simulink model "sampleModel7"  (R2021a)
settings: Solver=VariableStepAuto  StartTime=0.0  StopTime=10.0  RelTol=1e-3
undefined symbols (not defined in the file): DiscIntNeverNeededParam, magnitude, Newton, Raphson
libraries: simulink x210, pid_lib x47, simulink_need_slupdate x2
(part 5 of 8)

== system sampleModel7/cfblk409/cfblk12 ==
  cfblk1 : Inport
  cfblk11 : Inport  Port=2
  cfblk12 : Inport  Port=3
  cfblk13 : Inport  Port=4
  cfblk14 : Inport  Port=5
  cfblk10 : Constant  Value=[285971004.246024]  SampleTime=1
  cfblk3 : Delay  ShowEnablePort=on
      settings: InputPortMap=u0,e6
  cfblk4 : simulink/Discrete/Transfer Fcn Lead or Lag  PoleZ=0.95  ZeroZ=0.75  ICPrevOutput=0.0  ICPrevInput=0.0  DoSatur=off
      settings: SourceProductBaseCode=SL
  cfblk5 : Sum  Inputs=-+
  cfblk6 : MinMax  Function=max  Inputs=3
  cfblk7 : Rounding
  cfblk8 : Constant  Value=[956433965.581636]  SampleTime=1
  cfblk9 : Constant  Value=[825464940.183947]  SampleTime=1
  cfblk2 : Outport
  cfblk15 : Outport  Port=2
  wires:
  cfblk1/1 -> cfblk5/1
  cfblk12/1 -> cfblk15/1
  cfblk10/1 -> cfblk6/1
  cfblk7/1 -> cfblk5/2
  cfblk14/1 -> cfblk6/2
  cfblk13/1 -> cfblk6/3
  cfblk11/1 -> cfblk7/1
  cfblk9/1 -> cfblk3/1
  cfblk6/1 -> cfblk4/1
  cfblk5/1 -> cfblk3/2
  cfblk3/1 -> cfblk2/1

== system sampleModel7/cfblk410/cfblk6 ==
  cfblk1 : Inport
  cfblk9 : Inport  Port=2
  cfblk10 : Inport  Port=3
  cfblk11 : Inport  Port=4
  cfblk12 : Inport  Port=5
  cfblk3 : Product  Inputs=**
  cfblk4 : MinMax  Inputs=2
  cfblk5 : DotProduct  InputSameDT=on  OutDataTypeStr=Inherit: Inherit via internal rule
  cfblk6 : Constant  Value=[-599214719.429077]  SampleTime=1
  cfblk7 : Subsystem
  cfblk8 : Subsystem
  cfblk2 : Outport
  wires:
  cfblk11/1 -> cfblk5/1
  cfblk7/1(cfblk2) -> cfblk5/2
  cfblk5/1 -> cfblk8/1(cfblk1)
  cfblk6/1 -> cfblk2/1
  cfblk10/1 -> cfblk7/1(cfblk1), cfblk4/2
  cfblk3/1 -> cfblk7/2(cfblk13)
  cfblk9/1 -> cfblk3/1
  cfblk1/1 -> cfblk3/2
  cfblk12/1 -> cfblk8/2(cfblk7)
  cfblk8/1(cfblk2) -> cfblk4/1

== system sampleModel7/cfblk412/cfblk11 ==
  cfblk1 : Inport
  cfblk7 : Inport  Port=2
  cfblk8 : Inport  Port=3
  cfblk9 : Inport  Port=4
  cfblk3 : DiscreteFir
  cfblk4 : Sum  Inputs=|++
  cfblk5 : Rounding
  cfblk6 : Subsystem
  cfblk2 : Outport
  wires:
  cfblk3/1 -> cfblk4/1
  cfblk6/1(cfblk2) -> cfblk2/1
  cfblk8/1 -> cfblk4/2
  cfblk7/1 -> cfblk3/1
  cfblk5/1 -> cfblk6/1(cfblk1)
  cfblk1/1 -> cfblk6/2(cfblk12)
  cfblk9/1 -> cfblk5/1

== system sampleModel7/cfblk412/cfblk12 ==
  cfblk1 : Inport
  cfblk5 : Inport  Port=2
  cfblk6 : Inport  Port=3
  cfblk7 : Inport  Port=4
  cfblk8 : Inport  Port=5
  cfblk3 : simulink/Discrete/Tapped Delay  vinit=0.0  samptime=-1  NumDelays=1  DelayOrder=Oldest  includeCurrent=off
  cfblk4 : Gain  Gain=[760831877.903095]
  cfblk2 : Outport
  wires:
  cfblk1/1 -> cfblk3/1
  cfblk7/1 -> cfblk4/1
  cfblk3/1 -> cfblk2/1

== system sampleModel7/cfblk413/cfblk7 ==
  cfblk1 : Inport
  cfblk7 : Inport  Port=2
  cfblk8 : Inport  Port=3
  cfblk9 : Inport  Port=4
  cfblk10 : Inport  Port=5
  cfblk11 : Inport  Port=6
  cfblk12 : Inport  Port=7
  cfblk13 : Inport  Port=8
  cfblk3 : ComplexToRealImag
  cfblk4 : Gain  Gain=[-505145990.047614]
  cfblk5 : Product  Inputs=**
  cfblk6 : Assignment  DiagnosticForDimensions=Warning  IndexOptions=Index vector (dialog)  Indices=1  OutputSizes=1
  cfblk2 : Outport
  cfblk14 : Outport  Port=2
  wires:
  cfblk6/1 -> cfblk14/1
  cfblk11/1 -> cfblk3/1
  cfblk5/1 -> cfblk4/1
  cfblk9/1 -> cfblk5/1
  cfblk12/1 -> cfblk2/1
  cfblk3/1 -> cfblk6/1
  cfblk1/1 -> cfblk5/2
  cfblk8/1 -> cfblk6/2

== system sampleModel7/cfblk414/cfblk8 ==
  cfblk1 : Inport
  cfblk10 : Inport  Port=2
  cfblk11 : Inport  Port=3
  cfblk12 : Inport  Port=4
  cfblk13 : Inport  Port=5
  cfblk15 : Delay
  cfblk3 : DiscreteFir
  cfblk4 : Sum  Inputs=+
  cfblk5 : Product
  cfblk6 : Constant  Value=[-301322908.390573]  SampleTime=1
  cfblk7 : Constant  Value=[-743268385.761539]  SampleTime=1
  cfblk8 : Constant  Value=[952161668.056087]  SampleTime=1
  cfblk9 : Constant  Value=[508901382.821117]  SampleTime=1
  cfblk2 : Outport
  cfblk14 : Outport  Port=2
  wires:
  cfblk7/1 -> cfblk2/1
  cfblk9/1 -> cfblk14/1
  cfblk6/1 -> cfblk5/1
  cfblk3/1 -> cfblk5/2
  cfblk13/1 -> cfblk4/1
  cfblk5/1 -> cfblk15/1
  cfblk15/1 -> cfblk3/1

== system sampleModel7/cfblk347/cfblk15/cfblk17 ==
  cfblk1 : Inport
  cfblk11 : Inport  Port=2
  Action Port : ActionPort  ActionPortLabel=if(u1 >= 0)
  cfblk10 : Constant  Value=[-608024514.783165]  SampleTime=1
  cfblk12 : Delay
  cfblk3 : Delay  DelayLengthSource=Input port
      settings: InputPortMap=u0,p1
  cfblk4 : simulink/Discrete/Tapped Delay  vinit=0.0  samptime=-1  NumDelays=1  DelayOrder=Oldest  includeCurrent=off
  cfblk5 : DiscreteIntegrator  SampleTime=-1  ICPrevOutput=DiscIntNeverNeededParam  ICPrevScaledInput=DiscIntNeverNeededParam
  cfblk6 : Abs
  cfblk7 : Math  Operator=10^u  SaturateOnIntegerOverflow=on
  cfblk8 : Constant  Value=[523718034.088355]  SampleTime=1
  cfblk9 : Constant  Value=[-316304220.786418]  SampleTime=1
  cfblk2 : Outport
  wires:
  cfblk5/1 -> cfblk7/1
  cfblk4/1 -> cfblk3/1
  cfblk8/1 -> cfblk6/1
  cfblk6/1 -> cfblk3/2
  cfblk9/1 -> cfblk2/1
  cfblk11/1 -> cfblk4/1
  cfblk7/1 -> cfblk12/1
  cfblk12/1 -> cfblk5/1

== system sampleModel7/cfblk347/cfblk15/cfblk18 ==
  cfblk1 : Inport
  cfblk11 : Inport  Port=2
  cfblk12 : Inport  Port=3
  cfblk13 : Inport  Port=4
  cfblk14 : Inport  Port=5
  Action Port : ActionPort  ActionPortLabel=else
  cfblk10 : Product
  cfblk3 : simulink/Discrete/Transfer Fcn First Order  PoleZ=0.95  ICPrevOutput=0.0  DoSatur=off
  cfblk4 : simulink/Discrete/Transfer Fcn Real Zero  ZeroZ=0.75  ICPrevInput=0.0  DoSatur=off
      settings: SourceProductBaseCode=SL
  cfblk5 : Delay  DelayLengthSource=Input port
      settings: InputPortMap=u0,p1
  cfblk6 : simulink/Discrete/Difference  ICPrevInput=0.0  OutMin=[]  OutMax=[]  OutDataTypeStr=Inherit: Inherit via back propagation  OutDataType=fixdt(1, 16)  OutScaling=2^-10  DoSatur=off
  cfblk7 : ComplexToRealImag
  cfblk8 : Polyval  Coefs=[ +2.081618890e-019, -1.441693666e-014, +4.719686976e-010, -8.536869453e-006, +1.621573104e-001, -8.087801117e+001 ]
  cfblk9 : Trigonometry
  cfblk2 : Outport
  wires:
  cfblk10/1 -> cfblk2/1
  cfblk4/1 -> cfblk6/1
  cfblk8/1 -> cfblk3/1
  cfblk12/1 -> cfblk8/1
  cfblk7/1 -> cfblk10/1
  cfblk13/1 -> cfblk5/1
  cfblk9/1 -> cfblk7/1
  cfblk1/1 -> cfblk10/2
  cfblk14/1 -> cfblk5/2
  cfblk3/1 -> cfblk4/1
  cfblk5/1 -> cfblk9/1

== system sampleModel7/cfblk347/cfblk16/cfblk11 ==
  cfblk1 : Inport
  cfblk9 : Inport  Port=2
  cfblk10 : Inport  Port=3
  cfblk3 : simulink/Discrete/Transfer Fcn Lead or Lag  PoleZ=0.95  ZeroZ=0.75  ICPrevOutput=0.0  ICPrevInput=0.0  DoSatur=off
      settings: SourceProductBaseCode=SL
  cfblk4 : simulink/Discrete/Tapped Delay  vinit=0.0  samptime=-1  NumDelays=1  DelayOrder=Oldest  includeCurrent=off
  cfblk5 : UnaryMinus
  cfblk6 : simulink/Math Operations/MinMax Running Resettable  Function=min  vinit=0.0
  cfblk7 : Sqrt  SaturateOnIntegerOverflow=on
  cfblk8 : Constant  Value=[-882752696.159615]  SampleTime=1
  cfblk2 : Outport
  cfblk11 : Outport  Port=2
  wires:
  cfblk1/1 -> cfblk2/1
  cfblk6/1 -> cfblk3/1
  cfblk8/1 -> cfblk5/1
  cfblk9/1 -> cfblk6/1
  cfblk10/1 -> cfblk4/1
  cfblk5/1 -> cfblk6/2
  cfblk3/1 -> cfblk7/1
  cfblk7/1 -> cfblk11/1

== system sampleModel7/cfblk347/cfblk16/cfblk16 ==
  cfblk1 : Inport
  cfblk12 : Inport  Port=2
  cfblk13 : Inport  Port=3
  cfblk14 : Inport  Port=4
  cfblk15 : Inport  Port=5
  Action Port : ActionPort  ActionPortLabel=if(u1 >= 0)
  cfblk10 : Sin  TimeSource=Use external signal  SampleTime=0
  cfblk11 : Constant  Value=[176839491.235226]  SampleTime=1
  cfblk16 : Delay
  cfblk3 : DiscreteFilter
  cfblk4 : DiscreteTransferFcn
  cfblk5 : UnaryMinus
  cfblk6 : UnaryMinus
  cfblk7 : Sum  Inputs=+-
  cfblk8 : Trigonometry
  cfblk9 : Sum  Inputs=|++
  cfblk2 : Outport
  wires:
  cfblk13/1 -> cfblk6/1
  cfblk15/1 -> cfblk3/1
  cfblk9/1 -> cfblk8/1
  cfblk8/1 -> cfblk5/1
  cfblk12/1 -> cfblk4/1
  cfblk4/1 -> cfblk7/1
  cfblk3/1 -> cfblk10/1
  cfblk10/1 -> cfblk2/1
  cfblk6/1 -> cfblk7/2
  cfblk1/1 -> cfblk9/2
  cfblk5/1 -> cfblk16/1
  cfblk16/1 -> cfblk9/1

== system sampleModel7/cfblk347/cfblk16/cfblk17 ==
  cfblk1 : Inport
  cfblk10 : Inport  Port=2
  Action Port : ActionPort  ActionPortLabel=else
  cfblk3 : DiscreteFilter
  cfblk4 : DiscreteStateSpace  SampleTime=-1
  cfblk5 : simulink/Discrete/Transfer Fcn Real Zero  ZeroZ=0.75  ICPrevInput=0.0  DoSatur=off
      settings: SourceProductBaseCode=SL
  cfblk6 : Signum
  cfblk7 : DotProduct  InputSameDT=on  OutDataTypeStr=Inherit: Inherit via internal rule
  cfblk8 : Constant  Value=[-22627690.885052]  SampleTime=1
  cfblk9 : Constant  Value=[-586775164.786832]  SampleTime=1
  cfblk2 : Outport
  wires:
  cfblk1/1 -> cfblk7/1
  cfblk5/1 -> cfblk7/2
  cfblk4/1 -> cfblk3/1
  cfblk10/1 -> cfblk5/1
  cfblk8/1 -> cfblk4/1
  cfblk7/1 -> cfblk2/1
  cfblk9/1 -> cfblk6/1

== system sampleModel7/cfblk349/cfblk10/cfblk10 ==
  cfblk1 : Inport
  cfblk11 : Inport  Port=2
  cfblk12 : Inport  Port=3
  cfblk10 : Subsystem
  cfblk3 : DiscreteTransferFcn  SampleTime=1
  cfblk4 : DiscreteIntegrator  ICPrevOutput=DiscIntNeverNeededParam  ICPrevScaledInput=DiscIntNeverNeededParam
  cfblk5 : DiscreteIntegrator  ICPrevOutput=DiscIntNeverNeededParam  ICPrevScaledInput=DiscIntNeverNeededParam
  cfblk6 : Product
  cfblk7 : Product  Inputs=*
  cfblk8 : Squeeze
  cfblk9 : Constant  Value=[556466906.577604]  SampleTime=1
  cfblk2 : Outport
  wires:
  cfblk5/1 -> cfblk6/1
  cfblk11/1 -> cfblk2/1, cfblk10/3(cfblk16)
  cfblk9/1 -> cfblk3/1
  cfblk1/1 -> cfblk8/1
  cfblk12/1 -> cfblk5/1
  cfblk4/1 -> cfblk7/1, cfblk10/4(cfblk17)
  cfblk7/1 -> cfblk6/2
  cfblk3/1 -> cfblk4/1
  cfblk8/1 -> cfblk10/1(cfblk1)
  cfblk6/1 -> cfblk10/2(cfblk15)

== system sampleModel7/cfblk349/cfblk10/cfblk9 ==
  cfblk1 : Inport
  cfblk7 : Inport  Port=2
  cfblk3 : DiscreteTransferFcn  SampleTime=1
  cfblk4 : Bias  Bias=[918591324.613019]
  cfblk5 : Constant  Value=[221700069.480241]  SampleTime=1
  cfblk6 : Subsystem
  cfblk2 : Outport
  wires:
  cfblk4/1 -> cfblk2/1
  cfblk6/1(cfblk2) -> cfblk4/1
  cfblk5/1 -> cfblk3/1, cfblk6/4(cfblk10)
  cfblk3/1 -> cfblk6/1(cfblk1)
  cfblk7/1 -> cfblk6/2(cfblk8)
  cfblk1/1 -> cfblk6/3(cfblk9)

== system sampleModel7/cfblk350/cfblk13/cfblk10 ==
  cfblk1 : Inport
  cfblk6 : Inport  Port=2
  cfblk7 : Inport  Port=3
  cfblk3 : DiscreteFilter  SampleTime=1
  cfblk4 : Delay  SampleTime=1
  cfblk5 : Rounding
  cfblk2 : Outport
  wires:
  cfblk6/1 -> cfblk4/1
  cfblk4/1 -> cfblk5/1
  cfblk7/1 -> cfblk3/1
  cfblk5/1 -> cfblk2/1

== system sampleModel7/cfblk350/cfblk13/cfblk11 ==
  cfblk1 : Inport
  cfblk6 : Inport  Port=2
  cfblk7 : Inport  Port=3
  cfblk8 : Inport  Port=4
  cfblk9 : Inport  Port=5
  cfblk10 : Inport  Port=6
  cfblk11 : Inport  Port=7
  cfblk3 : DiscreteTransferFcn  SampleTime=1
  cfblk4 : simulink/Discrete/Tapped Delay  vinit=0.0  samptime=-1  NumDelays=1  DelayOrder=Oldest  includeCurrent=off
  cfblk5 : Reshape
  cfblk2 : Outport
  wires:
  cfblk6/1 -> cfblk3/1
  cfblk10/1 -> cfblk4/1
  cfblk8/1 -> cfblk2/1
  cfblk9/1 -> cfblk5/1

== system sampleModel7/cfblk350/cfblk13/cfblk16 ==
  cfblk1 : Inport
  cfblk13 : Inport  Port=2
  Action Port : ActionPort  ActionPortLabel=if(u1 >= 0)
  cfblk10 : Constant  Value=[-356294299.013930]  SampleTime=1
  cfblk11 : Constant  Value=[204123199.410798]  SampleTime=1
  cfblk12 : Subsystem
  cfblk3 : simulink/Discrete/Difference  ICPrevInput=0.0  OutMin=[]  OutMax=[]  OutDataTypeStr=Inherit: Inherit via back propagation  OutDataType=fixdt(1, 16)  OutScaling=2^-10  DoSatur=off
  cfblk4 : Bias  Bias=[30056507.447809]
  cfblk5 : UnaryMinus
  cfblk6 : Squeeze
  cfblk7 : Rounding
  cfblk8 : Trigonometry
  cfblk9 : Constant  Value=[-885448027.959644]  SampleTime=1
  cfblk2 : Outport
  wires:
  cfblk1/1 -> cfblk7/1
  cfblk5/1 -> cfblk12/1(cfblk1)
  cfblk4/1 -> cfblk5/1
  cfblk10/1 -> cfblk6/1
  cfblk3/1 -> cfblk2/1
  cfblk11/1 -> cfblk8/1
  cfblk9/1 -> cfblk12/2(cfblk8)
  cfblk7/1 -> cfblk3/1
  cfblk13/1 -> cfblk4/1
  cfblk8/1 -> cfblk12/3(cfblk9)

== system sampleModel7/cfblk350/cfblk13/cfblk17 ==
  cfblk1 : Inport
  cfblk7 : Inport  Port=2
  cfblk8 : Inport  Port=3
  cfblk9 : Inport  Port=4
  Action Port : ActionPort  ActionPortLabel=else
  cfblk10 : Delay
  cfblk11 : Delay
  cfblk3 : simulink/Discrete/Difference  ICPrevInput=0.0  OutMin=[]  OutMax=[]  OutDataTypeStr=Inherit: Inherit via back propagation  OutDataType=fixdt(1, 16)  OutScaling=2^-10  DoSatur=off
  cfblk4 : Signum
  cfblk5 : Subsystem
  cfblk6 : Subsystem
  cfblk2 : Outport
  wires:
  cfblk1/1 -> cfblk2/1
  cfblk3/1 -> cfblk4/1
  cfblk4/1 -> cfblk5/1(cfblk1)
  cfblk5/1(cfblk2) -> cfblk6/1(cfblk1)
  cfblk9/1 -> cfblk3/1
  cfblk7/1 -> cfblk6/2(cfblk14)
  cfblk8/1 -> cfblk6/3(cfblk15)
  cfblk6/1(cfblk2) -> cfblk10/1
  cfblk10/1 -> cfblk5/2(cfblk10)
  cfblk6/2(cfblk16) -> cfblk11/1
  cfblk11/1 -> cfblk5/3(cfblk11)

== system sampleModel7/cfblk351/cfblk8/cfblk7 ==
  cfblk1 : Inport
  cfblk9 : Inport  Port=2
  cfblk10 : Subsystem  TreatAsAtomicUnit=on
  cfblk11 : Subsystem  TreatAsAtomicUnit=on
  cfblk{12..16} (5 alike) : Delay  SampleTime=1
  cfblk3 : DiscreteFilter  SampleTime=1
  cfblk4 : Delay  ShowEnablePort=on  SampleTime=1
      settings: InputPortMap=u0,e6
  cfblk5 : DiscreteIntegrator  ICPrevOutput=DiscIntNeverNeededParam  ICPrevScaledInput=DiscIntNeverNeededParam
  cfblk6 : DotProduct  InputSameDT=on  OutDataTypeStr=Inherit: Inherit via internal rule
  cfblk7 : DotProduct  InputSameDT=on  OutDataTypeStr=Inherit: Inherit via internal rule
  cfblk8 : If  IfExpression=u1 >= 0  SampleTime=1
  cfblk2 : Outport
  wires:
  cfblk3/1 -> cfblk6/1, cfblk16/1
  cfblk7/1 -> cfblk10/1(cfblk1)
  cfblk10/1(cfblk2) -> cfblk3/1
  cfblk1/1 -> cfblk7/1, cfblk11/3(cfblk14)
  cfblk5/1 -> cfblk7/2
  cfblk6/1 -> cfblk12/1, cfblk13/1, cfblk14/1, cfblk15/1
  cfblk11/1(cfblk2) -> cfblk2/1
  cfblk9/1 -> cfblk4/1, cfblk4/2, cfblk11/4(cfblk15)
  cfblk10/2(cfblk13) -> cfblk6/2
  cfblk4/1 -> cfblk5/1
  cfblk8/1 -> cfblk10/Action
  cfblk8/2 -> cfblk11/Action
  cfblk12/1 -> cfblk11/1(cfblk1)
  cfblk13/1 -> cfblk10/2(cfblk11)
  cfblk14/1 -> cfblk11/2(cfblk13)
  cfblk15/1 -> cfblk10/3(cfblk12)
  cfblk16/1 -> cfblk8/1

== system sampleModel7/cfblk351/cfblk8/cfblk8 ==
  cfblk1 : Inport
  cfblk10 : Inport  Port=2
  cfblk11 : Inport  Port=3
  cfblk12 : Inport  Port=4
  cfblk13 : Inport  Port=5
  cfblk3 : simulink/Discrete/Transfer Fcn Lead or Lag  PoleZ=0.95  ZeroZ=0.75  ICPrevOutput=0.0  ICPrevInput=0.0  DoSatur=off
      settings: SourceProductBaseCode=SL
  cfblk4 : UnitDelay  HasFrameUpgradeWarning=on
  cfblk5 : Sum  Inputs=|++
  cfblk6 : Sqrt  SaturateOnIntegerOverflow=on
  cfblk7 : Constant  Value=[929234714.959824]  SampleTime=1
  cfblk8 : Constant  Value=[-420275551.072317]  SampleTime=1
  cfblk9 : Subsystem
  cfblk2 : Outport
  wires:
  cfblk7/1 -> cfblk4/1
  cfblk10/1 -> cfblk5/1
  cfblk11/1 -> cfblk2/1
  cfblk1/1 -> cfblk9/1(cfblk1)
  cfblk5/1 -> cfblk9/2(cfblk8)
  cfblk6/1 -> cfblk5/2
  cfblk9/1(cfblk2) -> cfblk3/1
  cfblk4/1 -> cfblk6/1

== system sampleModel7/cfblk353/cfblk8/cfblk11 ==
  cfblk1 : Inport
  cfblk8 : Inport  Port=2
  cfblk9 : Inport  Port=3
  cfblk3 : UnaryMinus
  cfblk4 : Constant  Value=[-773156934.291051]  SampleTime=1
  cfblk5 : Constant  Value=[763681732.988614]  SampleTime=1
  cfblk6 : Constant  Value=[876175884.597005]  SampleTime=1
  cfblk7 : Subsystem
  cfblk2 : Outport
  wires:
  cfblk4/1 -> cfblk7/1(cfblk1)
  cfblk1/1 -> cfblk3/1
  cfblk8/1 -> cfblk7/2(cfblk7)
  cfblk9/1 -> cfblk7/3(cfblk8)
  cfblk6/1 -> cfblk2/1
  cfblk5/1 -> cfblk7/4(cfblk9)
  cfblk3/1 -> cfblk7/5(cfblk10)

== system sampleModel7/cfblk354/cfblk18/cfblk11 ==
  cfblk1 : Inport
  cfblk9 : Inport  Port=2
  cfblk10 : Inport  Port=3
  cfblk11 : Inport  Port=4
  cfblk12 : Inport  Port=5
  cfblk13 : Inport  Port=6
  cfblk14 : Delay
  cfblk3 : DiscreteTransferFcn
  cfblk4 : Sin  TimeSource=Use external signal  SampleTime=0
  cfblk5 : Squeeze
  cfblk6 : Sqrt  Operator=rSqrt  AlgorithmType=Newton-Raphson  SaturateOnIntegerOverflow=on
  cfblk7 : Gain  Gain=[495087187.063231]
  cfblk8 : Subsystem
  cfblk2 : Outport
  wires:
  cfblk7/1 -> cfblk8/1(cfblk1)
  cfblk13/1 -> cfblk4/1
  cfblk10/1 -> cfblk6/1
  cfblk6/1 -> cfblk2/1
  cfblk5/1 -> cfblk7/1
  cfblk9/1 -> cfblk8/2(cfblk16)
  cfblk12/1 -> cfblk8/3(cfblk17)
  cfblk4/1 -> cfblk3/1
  cfblk8/1(cfblk2) -> cfblk14/1
  cfblk14/1 -> cfblk5/1

== system sampleModel7/cfblk354/cfblk18/cfblk15 ==
  cfblk1 : Inport
  cfblk11 : Inport  Port=2
  cfblk12 : Inport  Port=3
  Action Port : ActionPort  ActionPortLabel=if(u1 >= 0)
  cfblk10 : If  IfExpression=u1 >= 0  SampleTime=1
  cfblk13 : Subsystem  TreatAsAtomicUnit=on
  cfblk14 : Subsystem  TreatAsAtomicUnit=on
  cfblk{15..18} (4 alike) : Delay
  cfblk3 : pid_lib/PID Controller (2DOF)  Controller=PID  Form=Parallel  TimeDomain=Discrete-time  UseExternalTs=off  SampleTime=-1  IntegratorMethod=Forward Euler  FilterMethod=Forward Euler  ControllerParametersSource=internal  P=1  I=1  D=0  UseFilter=on  N=100  b=1  c=1  TunerSelectOption=Transfer Function Based (PID Tuner App)  InitialConditionSource=internal  InitialConditionForIntegrator=0  InitialConditionForFilter=0  DifferentiatorICPrevScaledInput=0  ExternalReset=none  TrackingMode=off  Kt=1  LimitOutput=off  SatLimitsSource=internal  UpperSaturationLimit=inf  LowerSaturationLimit=-inf  LinearizeAsGain=off  AntiWindupMode=none  Kb=1  POutMin=[]  POutMax=[]  IOutMin=[]  IOutMax=[]  DOutMin=[]  DOutMax=[]  NOutMin=[]  NOutMax=[]  bOutMin=[]  bOutMax=[]  cOutMin=[]  cOutMax=[]  SumOutMin=[]  SumOutMax=[]  SaturationOutMin=[]  SaturationOutMax=[]  PParamMin=[]  PParamMax=[]  IParamMin=[]  IParamMax=[]  DParamMin=[]  DParamMax=[]  NParamMin=[]  NParamMax=[]  bParamMin=[]  bParamMax=[]  cParamMin=[]  cParamMax=[]  KbParamMin=[]  KbParamMax=[]  KtParamMin=[]  KtParamMax=[]  KbOutMin=[]  KbOutMax=[]  KtOutMin=[]  KtOutMax=[]  IntegratorOutMin=[]  IntegratorOutMax=[]  FilterOutMin=[]  FilterOutMax=[]  SumI1OutMin=[]  SumI1OutMax=[]  SumI2OutMin=[]  SumI2OutMax=[]  SumI3OutMin=[]  SumI3OutMax=[]  SumI4OutMin=[]  SumI4OutMax=[]  SumDOutMin=[]  SumDOutMax=[]  Sum1OutMin=[]  Sum1OutMax=[]  Sum2OutMin=[]  Sum2OutMax=[]  Sum3OutMin=[]  Sum3OutMax=[]  DifferentiatorOutMin=[]  DifferentiatorOutMax=[]  FilterDiffOutCoefMin=[]  FilterDiffOutCoefMax=[]  ReciprocalOutMin=[]  ReciprocalOutMax=[]  SumDenOutMin=[]  SumDenOutMax=[]  SumNumOutMin=[]  SumNumOutMax=[]  DivideOutMin=[]  DivideOutMax=[]  UdiffTsProdOutMin=[]  UdiffTsProdOutMax=[]  NTsProdOutMin=[]  NTsProdOutMax=[]  UintegralTsProdOutMin=[]  UintegralTsProdOutMax=[]  UngainTsProdOutMin=[]  UngainTsProdOutMax=[]  IntegratorContinuousStateAttributes=''  IntegratorStateMustResolveToSignalObject=off  IntegratorRTWStateStorageClass=Auto  FilterContinuousStateAttributes=''  FilterStateMustResolveToSignalObject=off  FilterRTWStateStorageClass=Auto  ParallelPVariant=InternalParameters  IdealPVariant=Disabled  IVariant=InternalParameters  DVariant=InternalParameters  bVariant=InternalParameters  cVariant=InternalParameters  IntegratorVariant=Discrete  SatVariant=Disabled  AWVariant=Passthrough  PCopyVariant=Disabled  TRVariant=Disabled  FdbkBlocksVariant=Forward  IdealPFdbkVariant=Disabled  SatFdbkVariant=Disabled  DerivativeFilterVariant=ForwardEulerFilter  NVariant=InternalParameters  NCopyVariant=Disabled  FilterICVariant=InternalICsFilter  IntegratorICVariant=InternalICs  ExternalResetVariant=Disabled  TRSumVariant=Passthrough  SumFdbkVariant=Disabled  SumVariant=Sum_PID  TsampFilterVariant=InternalTs  TsampNgainVariant=Passthrough  TsampIntegralVariant=Passthrough  ExternalSaturationOutDataTypeStr=Inherit: Same as second input
      settings: SourceProductBaseCode=SL
  cfblk4 : DiscreteZeroPole  Poles=[0 0.5]  Gain=1  SampleTime=-1
  cfblk5 : UnitDelay  SampleTime=-1  HasFrameUpgradeWarning=on
  cfblk6 : simulink/Discrete/Tapped Delay  vinit=0.0  samptime=-1  NumDelays=1  DelayOrder=Oldest  includeCurrent=off
  cfblk7 : ComplexToMagnitudeAngle
  cfblk8 : Constant  Value=[-929461708.025462]  SampleTime=1
  cfblk9 : Constant  Value=[369701314.972565]  SampleTime=1
  cfblk2 : Outport
  wires:
  cfblk14/1(cfblk2) -> cfblk3/1
  cfblk1/1 -> cfblk14/1(cfblk1)
  cfblk13/1(cfblk2) -> cfblk7/1
  cfblk11/1 -> cfblk14/2(cfblk11)
  cfblk9/1 -> cfblk5/1
  cfblk7/1 -> cfblk2/1
  cfblk5/1 -> cfblk10/1
  cfblk4/1 -> cfblk6/1, cfblk17/1
  cfblk8/1 -> cfblk3/2, cfblk14/4(cfblk13), cfblk14/5(cfblk14)
  cfblk3/1 -> cfblk4/1, cfblk18/1
  cfblk12/1 -> cfblk13/2(cfblk7)
  cfblk10/1 -> cfblk13/Action
  cfblk10/2 -> cfblk14/Action
  cfblk6/1 -> cfblk15/1
  cfblk15/1 -> cfblk13/3(cfblk8)
  cfblk7/2 -> cfblk16/1
  cfblk16/1 -> cfblk13/1(cfblk1)
  cfblk17/1 -> cfblk13/4(cfblk9)
  cfblk18/1 -> cfblk14/3(cfblk12)

== system sampleModel7/cfblk354/cfblk18/cfblk16 ==
  cfblk1 : Inport
  Action Port : ActionPort  ActionPortLabel=else
  cfblk10 : Subsystem  TreatAsAtomicUnit=on
  cfblk11 : Subsystem  TreatAsAtomicUnit=on
  cfblk12 : Delay
  cfblk3 : simulink/Discrete/Difference  ICPrevInput=0.0  OutMin=[]  OutMax=[]  OutDataTypeStr=Inherit: Inherit via back propagation  OutDataType=fixdt(1, 16)  OutScaling=2^-10  DoSatur=off
  cfblk4 : Delay  DelayLengthSource=Input port
      settings: InputPortMap=u0,p1
  cfblk5 : Gain  Gain=[449671895.081217]
  cfblk6 : ComplexToMagnitudeAngle
  cfblk7 : Constant  Value=[495584420.253082]  SampleTime=1
  cfblk8 : Constant  Value=[-455781378.164525]  SampleTime=1
  cfblk9 : If  IfExpression=u1 >= 0  SampleTime=1
  cfblk2 : Outport
  wires:
  cfblk3/1 -> cfblk5/1
  cfblk8/1 -> cfblk10/1(cfblk1)
  cfblk6/1 -> cfblk3/1
  cfblk11/1(cfblk2) -> cfblk4/1
  cfblk4/1 -> cfblk2/1
  cfblk6/2 -> cfblk4/2
  cfblk1/1 -> cfblk10/2(cfblk8), cfblk11/3(cfblk12)
  cfblk10/1(cfblk2) -> cfblk6/1
  cfblk10/2(cfblk9) -> cfblk11/1(cfblk1)
  cfblk7/1 -> cfblk11/2(cfblk11)
  cfblk9/1 -> cfblk10/Action
  cfblk9/2 -> cfblk11/Action
  cfblk5/1 -> cfblk12/1
  cfblk12/1 -> cfblk9/1

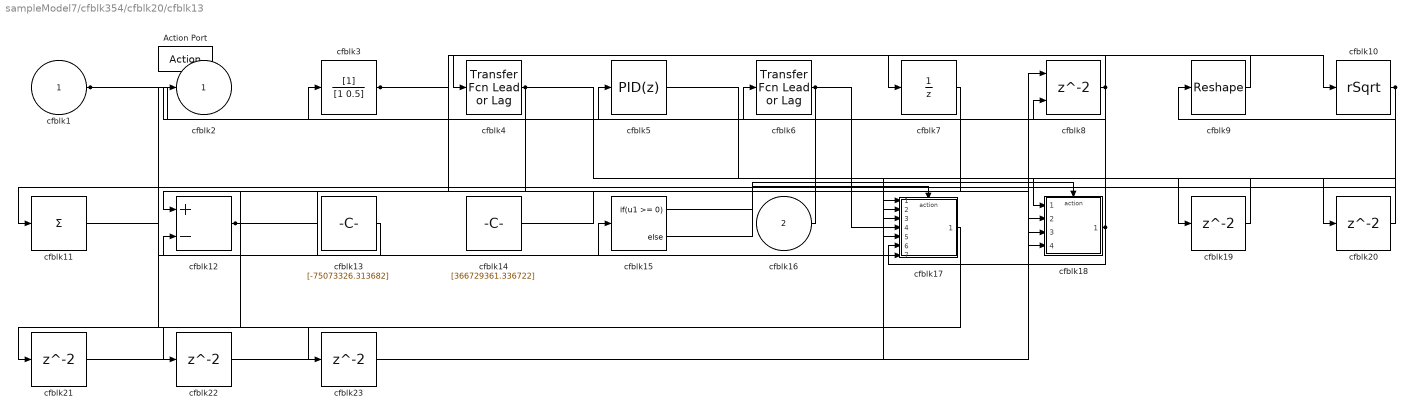
== system sampleModel7/cfblk354/cfblk20/cfblk13 ==
  cfblk1 : Inport
  cfblk16 : Inport  Port=2
  Action Port : ActionPort  ActionPortLabel=if(u1 >= 0)
  cfblk10 : Sqrt  Operator=rSqrt  AlgorithmType=Newton-Raphson  SaturateOnIntegerOverflow=on
  cfblk11 : Sum  Inputs=+
  cfblk12 : Sum  Inputs=+-
  cfblk13 : Constant  Value=[-75073326.313682]  SampleTime=1
  cfblk14 : Constant  Value=[366729361.336722]  SampleTime=1
  cfblk15 : If  IfExpression=u1 >= 0  SampleTime=1
  cfblk17 : Subsystem  TreatAsAtomicUnit=on
  cfblk18 : Subsystem  TreatAsAtomicUnit=on
  cfblk{19..23} (5 alike) : Delay
  cfblk3 : DiscreteFilter
  cfblk4 : simulink/Discrete/Transfer Fcn Lead or Lag  PoleZ=0.95  ZeroZ=0.75  ICPrevOutput=0.0  ICPrevInput=0.0  DoSatur=off
      settings: SourceProductBaseCode=SL
  cfblk5 : pid_lib/PID Controller  Controller=PID  Form=Parallel  TimeDomain=Discrete-time  UseExternalTs=off  SampleTime=-1  IntegratorMethod=Forward Euler  FilterMethod=Forward Euler  ControllerParametersSource=internal  P=1  I=1  D=0  UseFilter=on  N=100  TunerSelectOption=Transfer Function Based (PID Tuner App)  InitialConditionSource=internal  InitialConditionForIntegrator=0  InitialConditionForFilter=0  DifferentiatorICPrevScaledInput=0  ExternalReset=none  TrackingMode=off  Kt=1  LimitOutput=off  SatLimitsSource=internal  UpperSaturationLimit=inf  LowerSaturationLimit=-inf  LinearizeAsGain=off  AntiWindupMode=none  Kb=1  POutMin=[]  POutMax=[]  IOutMin=[]  IOutMax=[]  DOutMin=[]  DOutMax=[]  NOutMin=[]  NOutMax=[]  SumOutMin=[]  SumOutMax=[]  SaturationOutMin=[]  SaturationOutMax=[]  PParamMin=[]  PParamMax=[]  IParamMin=[]  IParamMax=[]  DParamMin=[]  DParamMax=[]  NParamMin=[]  NParamMax=[]  KbParamMin=[]  KbParamMax=[]  KtParamMin=[]  KtParamMax=[]  KbOutMin=[]  KbOutMax=[]  KtOutMin=[]  KtOutMax=[]  IntegratorOutMin=[]  IntegratorOutMax=[]  FilterOutMin=[]  FilterOutMax=[]  SumI1OutMin=[]  SumI1OutMax=[]  SumI2OutMin=[]  SumI2OutMax=[]  SumI3OutMin=[]  SumI3OutMax=[]  SumI4OutMin=[]  SumI4OutMax=[]  SumDOutMin=[]  SumDOutMax=[]  DifferentiatorOutMin=[]  DifferentiatorOutMax=[]  FilterDiffOutCoefMin=[]  FilterDiffOutCoefMax=[]  ReciprocalOutMin=[]  ReciprocalOutMax=[]  SumDenOutMin=[]  SumDenOutMax=[]  SumNumOutMin=[]  SumNumOutMax=[]  DivideOutMin=[]  DivideOutMax=[]  UdiffTsProdOutMin=[]  UdiffTsProdOutMax=[]  NTsProdOutMin=[]  NTsProdOutMax=[]  UintegralTsProdOutMin=[]  UintegralTsProdOutMax=[]  UngainTsProdOutMin=[]  UngainTsProdOutMax=[]  IntegratorContinuousStateAttributes=''  IntegratorStateMustResolveToSignalObject=off  IntegratorRTWStateStorageClass=Auto  FilterContinuousStateAttributes=''  FilterStateMustResolveToSignalObject=off  FilterRTWStateStorageClass=Auto  ParallelPVariant=InternalParameters  IdealPVariant=Disabled  IVariant=InternalParameters  DVariant=InternalParameters  IntegratorVariant=Discrete  SatVariant=Disabled  AWVariant=Passthrough  PCopyVariant=Disabled  TRVariant=Disabled  FdbkBlocksVariant=Forward  IdealPFdbkVariant=Disabled  SatFdbkVariant=Disabled  DerivativeFilterVariant=ForwardEulerFilter  NVariant=InternalParameters  NCopyVariant=Disabled  FilterICVariant=InternalICsFilter  IntegratorICVariant=InternalICs  ExternalResetVariant=Disabled  TRSumVariant=Passthrough  SumFdbkVariant=Disabled  SumVariant=Sum_PID  TsampFilterVariant=InternalTs  TsampNgainVariant=Passthrough  TsampIntegralVariant=Passthrough  ExternalSaturationOutDataTypeStr=Inherit: Same as second input
  cfblk6 : simulink/Discrete/Transfer Fcn Lead or Lag  PoleZ=0.95  ZeroZ=0.75  ICPrevOutput=0.0  ICPrevInput=0.0  DoSatur=off
      settings: SourceProductBaseCode=SL
  cfblk7 : UnitDelay  SampleTime=-1  HasFrameUpgradeWarning=on
  cfblk8 : Delay  ShowEnablePort=on
      settings: InputPortMap=u0,e6
  cfblk9 : Reshape
  cfblk2 : Outport
  wires:
  cfblk8/1 -> cfblk4/1, cfblk11/1
  cfblk7/1 -> cfblk12/1
  cfblk1/1 -> cfblk3/1, cfblk17/7(cfblk14)
  cfblk16/1 -> cfblk6/1
  cfblk12/1 -> cfblk15/1, cfblk17/3(cfblk10)
  cfblk13/1 -> cfblk12/2
  cfblk9/1 -> cfblk7/1
  cfblk10/1 -> cfblk9/1, cfblk18/4(cfblk17)
  cfblk6/1 -> cfblk2/1, cfblk17/4(cfblk11)
  cfblk14/1 -> cfblk18/2(cfblk15)
  cfblk18/1(cfblk2) -> cfblk5/1, cfblk8/2, cfblk17/6(cfblk13)
  cfblk3/1 -> cfblk18/3(cfblk16), cfblk10/1
  cfblk4/1 -> cfblk20/1, cfblk22/1
  cfblk15/1 -> cfblk17/Action
  cfblk15/2 -> cfblk18/Action
  cfblk5/1 -> cfblk19/1
  cfblk19/1 -> cfblk18/1(cfblk1)
  cfblk20/1 -> cfblk17/2(cfblk9)
  cfblk17/1(cfblk2) -> cfblk21/1
  cfblk21/1 -> cfblk8/1
  cfblk22/1 -> cfblk17/5(cfblk12)
  cfblk11/1 -> cfblk23/1
  cfblk23/1 -> cfblk17/1(cfblk1)

== system sampleModel7/cfblk354/cfblk20/cfblk14 ==
  cfblk1 : Inport
  cfblk15 : Inport  Port=2
  cfblk16 : Inport  Port=3
  cfblk17 : Inport  Port=4
  Action Port : ActionPort  ActionPortLabel=else
  cfblk10 : Sum  Inputs=+
  cfblk11 : MinMax  Function=max
  cfblk12 : Sum  Inputs=+
  cfblk13 : Constant  Value=[-740044020.025766]  SampleTime=1
  cfblk14 : Constant  Value=[876341486.325344]  SampleTime=1
  cfblk18 : Delay
  cfblk3 : Delay  ShowEnablePort=on
      settings: InputPortMap=u0,e6
  cfblk4 : DiscreteZeroPole  Poles=[0 0.5]  Gain=1  SampleTime=-1
  cfblk5 : DiscreteStateSpace  SampleTime=-1
  cfblk6 : simulink/Discrete/Tapped Delay  vinit=0.0  samptime=-1  NumDelays=1  DelayOrder=Oldest  includeCurrent=off
  cfblk7 : DotProduct  InputSameDT=on  OutDataTypeStr=Inherit: Inherit via internal rule
  cfblk8 : Gain  Gain=[916469674.030527]
  cfblk9 : Assignment  DiagnosticForDimensions=Warning  IndexOptions=Index vector (dialog)  Indices=1  OutputSizes=1
  cfblk2 : Outport
  wires:
  cfblk16/1 -> cfblk12/1
  cfblk9/1 -> cfblk5/1
  cfblk5/1 -> cfblk8/1
  cfblk12/1 -> cfblk6/1
  cfblk7/1 -> cfblk10/1
  cfblk4/1 -> cfblk9/1
  cfblk15/1 -> cfblk9/2
  cfblk17/1 -> cfblk4/1
  cfblk14/1 -> cfblk3/1
  cfblk1/1 -> cfblk2/1
  cfblk3/1 -> cfblk11/1
  cfblk11/1 -> cfblk7/2
  cfblk6/1 -> cfblk3/2
  cfblk10/1 -> cfblk18/1
  cfblk18/1 -> cfblk7/1

== system sampleModel7/cfblk354/cfblk20/cfblk9 ==
  cfblk1 : Inport
  cfblk9 : Inport  Port=2
  cfblk10 : Inport  Port=3
  cfblk3 : DiscreteStateSpace  SampleTime=-1
  cfblk4 : PermuteDimensions
  cfblk5 : Squeeze
  cfblk6 : Polyval  Coefs=[ +2.081618890e-019, -1.441693666e-014, +4.719686976e-010, -8.536869453e-006, +1.621573104e-001, -8.087801117e+001 ]
  cfblk7 : Product  Inputs=*
  cfblk8 : Constant  Value=[-617028440.656956]  SampleTime=1
  cfblk2 : Outport
  wires:
  cfblk3/1 -> cfblk5/1
  cfblk9/1 -> cfblk3/1
  cfblk1/1 -> cfblk2/1
  cfblk8/1 -> cfblk4/1
  cfblk7/1 -> cfblk6/1
  cfblk5/1 -> cfblk7/1

== system sampleModel7/cfblk362/cfblk10/cfblk16 ==
  cfblk1 : Inport
  cfblk12 : Inport  Port=2
  cfblk13 : Inport  Port=3
  cfblk14 : Inport  Port=4
  cfblk15 : Inport  Port=5
  Action Port : ActionPort  ActionPortLabel=if(u1 >= 0)
  cfblk10 : Sin  TimeSource=Use external signal  SampleTime=0
  cfblk11 : Rounding
  cfblk3 : Delay  DelayLengthSource=Input port
      settings: InputPortMap=u0,p1
  cfblk4 : UnitDelay  SampleTime=-1  HasFrameUpgradeWarning=on
  cfblk5 : DiscreteFilter
  cfblk6 : PermuteDimensions
  cfblk7 : Sum  Inputs=+
  cfblk8 : Product  Inputs=**
  cfblk9 : Signum
  cfblk2 : Outport
  wires:
  cfblk15/1 -> cfblk10/1
  cfblk10/1 -> cfblk6/1
  cfblk7/1 -> cfblk5/1
  cfblk11/1 -> cfblk4/1
  cfblk6/1 -> cfblk8/1
  cfblk8/1 -> cfblk7/1
  cfblk14/1 -> cfblk8/2
  cfblk3/1 -> cfblk11/1
  cfblk13/1 -> cfblk9/1
  cfblk12/1 -> cfblk2/1
  cfblk5/1 -> cfblk3/1
  cfblk1/1 -> cfblk3/2

== system sampleModel7/cfblk362/cfblk10/cfblk17 ==
  cfblk1 : Inport
  cfblk7 : Inport  Port=2
  cfblk8 : Inport  Port=3
  Action Port : ActionPort  ActionPortLabel=else
  cfblk3 : Delay
  cfblk4 : Delay  ShowEnablePort=on
      settings: InputPortMap=u0,e6
  cfblk5 : simulink/Discrete/Transfer Fcn Lead or Lag  PoleZ=0.95  ZeroZ=0.75  ICPrevOutput=0.0  ICPrevInput=0.0  DoSatur=off
      settings: SourceProductBaseCode=SL
  cfblk6 : Constant  Value=[-590372430.966452]  SampleTime=1
  cfblk2 : Outport
  wires:
  cfblk8/1 -> cfblk4/1
  cfblk3/1 -> cfblk5/1
  cfblk4/1 -> cfblk2/1
  cfblk1/1 -> cfblk4/2
  cfblk6/1 -> cfblk3/1

== system sampleModel7/cfblk362/cfblk11/cfblk10 ==
  cfblk1 : Inport
  cfblk15 : Inport  Port=2
  cfblk16 : Inport  Port=3
  cfblk17 : Inport  Port=4
  cfblk10 : Constant  Value=[-2387252.625086]  SampleTime=1
  cfblk11 : Constant  Value=[-263113663.898132]  SampleTime=1
  cfblk12 : Subsystem
  cfblk13 : Subsystem
  cfblk14 : Subsystem
  cfblk18 : Delay
  cfblk3 : pid_lib/PID Controller (2DOF)  Controller=PID  Form=Parallel  TimeDomain=Discrete-time  UseExternalTs=off  SampleTime=-1  IntegratorMethod=Forward Euler  FilterMethod=Forward Euler  ControllerParametersSource=internal  P=1  I=1  D=0  UseFilter=on  N=100  b=1  c=1  TunerSelectOption=Transfer Function Based (PID Tuner App)  InitialConditionSource=internal  InitialConditionForIntegrator=0  InitialConditionForFilter=0  DifferentiatorICPrevScaledInput=0  ExternalReset=none  TrackingMode=off  Kt=1  LimitOutput=off  SatLimitsSource=internal  UpperSaturationLimit=inf  LowerSaturationLimit=-inf  LinearizeAsGain=off  AntiWindupMode=none  Kb=1  POutMin=[]  POutMax=[]  IOutMin=[]  IOutMax=[]  DOutMin=[]  DOutMax=[]  NOutMin=[]  NOutMax=[]  bOutMin=[]  bOutMax=[]  cOutMin=[]  cOutMax=[]  SumOutMin=[]  SumOutMax=[]  SaturationOutMin=[]  SaturationOutMax=[]  PParamMin=[]  PParamMax=[]  IParamMin=[]  IParamMax=[]  DParamMin=[]  DParamMax=[]  NParamMin=[]  NParamMax=[]  bParamMin=[]  bParamMax=[]  cParamMin=[]  cParamMax=[]  KbParamMin=[]  KbParamMax=[]  KtParamMin=[]  KtParamMax=[]  KbOutMin=[]  KbOutMax=[]  KtOutMin=[]  KtOutMax=[]  IntegratorOutMin=[]  IntegratorOutMax=[]  FilterOutMin=[]  FilterOutMax=[]  SumI1OutMin=[]  SumI1OutMax=[]  SumI2OutMin=[]  SumI2OutMax=[]  SumI3OutMin=[]  SumI3OutMax=[]  SumI4OutMin=[]  SumI4OutMax=[]  SumDOutMin=[]  SumDOutMax=[]  Sum1OutMin=[]  Sum1OutMax=[]  Sum2OutMin=[]  Sum2OutMax=[]  Sum3OutMin=[]  Sum3OutMax=[]  DifferentiatorOutMin=[]  DifferentiatorOutMax=[]  FilterDiffOutCoefMin=[]  FilterDiffOutCoefMax=[]  ReciprocalOutMin=[]  ReciprocalOutMax=[]  SumDenOutMin=[]  SumDenOutMax=[]  SumNumOutMin=[]  SumNumOutMax=[]  DivideOutMin=[]  DivideOutMax=[]  UdiffTsProdOutMin=[]  UdiffTsProdOutMax=[]  NTsProdOutMin=[]  NTsProdOutMax=[]  UintegralTsProdOutMin=[]  UintegralTsProdOutMax=[]  UngainTsProdOutMin=[]  UngainTsProdOutMax=[]  IntegratorContinuousStateAttributes=''  IntegratorStateMustResolveToSignalObject=off  IntegratorRTWStateStorageClass=Auto  FilterContinuousStateAttributes=''  FilterStateMustResolveToSignalObject=off  FilterRTWStateStorageClass=Auto  ParallelPVariant=InternalParameters  IdealPVariant=Disabled  IVariant=InternalParameters  DVariant=InternalParameters  bVariant=InternalParameters  cVariant=InternalParameters  IntegratorVariant=Discrete  SatVariant=Disabled  AWVariant=Passthrough  PCopyVariant=Disabled  TRVariant=Disabled  FdbkBlocksVariant=Forward  IdealPFdbkVariant=Disabled  SatFdbkVariant=Disabled  DerivativeFilterVariant=ForwardEulerFilter  NVariant=InternalParameters  NCopyVariant=Disabled  FilterICVariant=InternalICsFilter  IntegratorICVariant=InternalICs  ExternalResetVariant=Disabled  TRSumVariant=Passthrough  SumFdbkVariant=Disabled  SumVariant=Sum_PID  TsampFilterVariant=InternalTs  TsampNgainVariant=Passthrough  TsampIntegralVariant=Passthrough  ExternalSaturationOutDataTypeStr=Inherit: Same as second input
      settings: SourceProductBaseCode=SL
  cfblk4 : Sum  Inputs=+
  cfblk5 : Signum
  cfblk6 : Sum  Inputs=-+
  cfblk7 : Signum
  cfblk8 : ComplexToMagnitudeAngle
  cfblk9 : Constant  Value=[-313984426.676796]  SampleTime=1
  cfblk2 : Outport
  wires:
  cfblk16/1 -> cfblk3/1
  cfblk12/1(cfblk2) -> cfblk7/1
  cfblk13/1(cfblk2) -> cfblk4/1
  cfblk1/1 -> cfblk3/2
  cfblk11/1 -> cfblk8/1
  cfblk3/1 -> cfblk13/2(cfblk9)
  cfblk15/1 -> cfblk5/1
  cfblk5/1 -> cfblk12/1(cfblk1)
  cfblk4/1 -> cfblk14/1(cfblk1)
  cfblk7/1 -> cfblk2/1
  cfblk9/1 -> cfblk14/2(cfblk8)
  cfblk10/1 -> cfblk14/3(cfblk9)
  cfblk8/1 -> cfblk14/4(cfblk10)
  cfblk8/2 -> cfblk6/1
  cfblk14/1(cfblk2) -> cfblk6/2
  cfblk6/1 -> cfblk18/1
  cfblk18/1 -> cfblk13/1(cfblk1)

== system sampleModel7/cfblk362/cfblk6/cfblk17 ==
  cfblk1 : Inport
  cfblk7 : Inport  Port=2
  Action Port : ActionPort  ActionPortLabel=if(u1 >= 0)
  cfblk3 : Reshape
  cfblk4 : Sum  Inputs=+
  cfblk5 : Rounding
  cfblk6 : Constant  Value=[-18782019.800058]  SampleTime=1
  cfblk2 : Outport
  wires:
  cfblk1/1 -> cfblk2/1
  cfblk6/1 -> cfblk5/1
  cfblk5/1 -> cfblk4/1
  cfblk7/1 -> cfblk3/1

== system sampleModel7/cfblk362/cfblk6/cfblk18 ==
  cfblk1 : Inport
  cfblk11 : Inport  Port=2
  cfblk12 : Inport  Port=3
  cfblk13 : Inport  Port=4
  Action Port : ActionPort  ActionPortLabel=else
  cfblk10 : Constant  Value=[-791962928.687818]  SampleTime=1
  cfblk3 : simulink/Discrete/Transfer Fcn First Order  PoleZ=0.95  ICPrevOutput=0.0  DoSatur=off
  cfblk4 : DiscreteStateSpace  SampleTime=-1
  cfblk5 : simulink/Discrete/Transfer Fcn Real Zero  ZeroZ=0.75  ICPrevInput=0.0  DoSatur=off
      settings: SourceProductBaseCode=SL
  cfblk6 : DiscreteFir
  cfblk7 : Reshape
  cfblk8 : MinMax
  cfblk9 : PermuteDimensions
  cfblk2 : Outport
  wires:
  cfblk4/1 -> cfblk8/1
  cfblk9/1 -> cfblk2/1
  cfblk13/1 -> cfblk6/1
  cfblk5/1 -> cfblk3/1
  cfblk12/1 -> cfblk9/1
  cfblk6/1 -> cfblk5/1
  cfblk3/1 -> cfblk7/1
  cfblk1/1 -> cfblk4/1

== system sampleModel7/cfblk364/cfblk6/cfblk16 ==
  cfblk1 : Inport
  cfblk7 : Inport  Port=2
  Action Port : ActionPort  ActionPortLabel=if(u1 >= 0)
  cfblk3 : ComplexToRealImag
  cfblk4 : Subsystem
  cfblk5 : Subsystem
  cfblk6 : Subsystem
  cfblk8 : Delay
  cfblk9 : Delay
  cfblk2 : Outport
  wires:
  cfblk5/1(cfblk2) -> cfblk2/1, cfblk9/1
  cfblk7/1 -> cfblk6/1(cfblk1), cfblk4/6(cfblk14)
  cfblk1/1 -> cfblk3/1
  cfblk4/1(cfblk2) -> cfblk6/2(cfblk7), cfblk5/2(cfblk15)
  cfblk3/1 -> cfblk4/2(cfblk10)
  cfblk3/2 -> cfblk5/1(cfblk1), cfblk4/3(cfblk11), cfblk5/3(cfblk16), cfblk4/5(cfblk13)
  cfblk6/1(cfblk2) -> cfblk8/1
  cfblk8/1 -> cfblk4/1(cfblk1)
  cfblk9/1 -> cfblk4/4(cfblk12)

== system sampleModel7/cfblk364/cfblk6/cfblk17 ==
  cfblk1 : Inport
  Action Port : ActionPort  ActionPortLabel=else
  cfblk10 : Delay
  cfblk11 : Delay
  cfblk3 : simulink/Discrete/Transfer Fcn Real Zero  ZeroZ=0.75  ICPrevInput=0.0  DoSatur=off
      settings: SourceProductBaseCode=SL
  cfblk4 : Squeeze
  cfblk5 : Trigonometry
  cfblk6 : DotProduct  InputSameDT=on  OutDataTypeStr=Inherit: Inherit via internal rule
  cfblk7 : simulink/Math Operations/MinMax Running Resettable  Function=min  vinit=0.0
  cfblk8 : Trigonometry
  cfblk9 : Sum
  cfblk2 : Outport
  wires:
  cfblk6/1 -> cfblk9/1
  cfblk3/1 -> cfblk6/2, cfblk10/1
  cfblk1/1 -> cfblk7/2, cfblk6/1
  cfblk9/1 -> cfblk8/1
  cfblk8/1 -> cfblk4/1, cfblk5/1
  cfblk4/1 -> cfblk2/1
  cfblk7/1 -> cfblk3/1
  cfblk10/1 -> cfblk7/1
  cfblk5/1 -> cfblk11/1
  cfblk11/1 -> cfblk9/2

== system sampleModel7/cfblk364/cfblk6/cfblk18 ==
  cfblk1 : Inport
  cfblk8 : Inport  Port=2
  Action Port : ActionPort  ActionPortLabel=if(u1 >= 0)
  cfblk3 : Gain  Gain=[899471295.688868]
  cfblk4 : UnaryMinus
  cfblk5 : Bias  Bias=[554681337.672858]
  cfblk6 : Abs
  cfblk7 : Constant  Value=[361963143.280026]  SampleTime=1
  cfblk2 : Outport
  wires:
  cfblk6/1 -> cfblk5/1
  cfblk4/1 -> cfblk2/1
  cfblk1/1 -> cfblk3/1
  cfblk3/1 -> cfblk6/1
  cfblk5/1 -> cfblk4/1

== system sampleModel7/cfblk364/cfblk6/cfblk19 ==
  cfblk1 : Inport
  cfblk9 : Inport  Port=2
  cfblk10 : Inport  Port=3
  cfblk11 : Inport  Port=4
  cfblk12 : Inport  Port=5
  cfblk13 : Inport  Port=6
  Action Port : ActionPort  ActionPortLabel=else
  cfblk3 : Delay  DelayLengthSource=Input port
      settings: InputPortMap=u0,p1
  cfblk4 : UnaryMinus
  cfblk5 : Math  Operator=conj  SaturateOnIntegerOverflow=on
  cfblk6 : Sin  TimeSource=Use external signal  SampleTime=0
  cfblk7 : Constant  Value=[482103381.275899]  SampleTime=1
  cfblk8 : Constant  Value=[486945171.823239]  SampleTime=1
  cfblk2 : Outport
  wires:
  cfblk3/1 -> cfblk5/1
  cfblk11/1 -> cfblk3/1
  cfblk5/1 -> cfblk2/1
  cfblk9/1 -> cfblk3/2
  cfblk8/1 -> cfblk6/1
  cfblk12/1 -> cfblk4/1

== system sampleModel7/cfblk382/cfblk17/cfblk13 ==
  cfblk1 : Inport
  cfblk7 : Inport  Port=2
  Action Port : ActionPort  ActionPortLabel=if(u1 >= 0)
  cfblk3 : DiscreteZeroPole  Poles=[0 0.5]  Gain=1  SampleTime=-1
  cfblk4 : Sqrt  SaturateOnIntegerOverflow=on
  cfblk5 : Polyval  Coefs=[ +2.081618890e-019, -1.441693666e-014, +4.719686976e-010, -8.536869453e-006, +1.621573104e-001, -8.087801117e+001 ]
  cfblk6 : Subsystem
  cfblk8 : Delay
  cfblk2 : Outport
  wires:
  cfblk4/1 -> cfblk5/1
  cfblk1/1 -> cfblk3/1, cfblk6/3(cfblk8)
  cfblk6/1(cfblk2) -> cfblk2/1
  cfblk7/1 -> cfblk6/1(cfblk1)
  cfblk3/1 -> cfblk6/2(cfblk7)
  cfblk5/1 -> cfblk8/1
  cfblk8/1 -> cfblk4/1

== system sampleModel7/cfblk382/cfblk17/cfblk14 ==
  cfblk1 : Inport
  cfblk10 : Inport  Port=2
  cfblk11 : Inport  Port=3
  cfblk12 : Inport  Port=4
  Action Port : ActionPort  ActionPortLabel=else
  cfblk13 : Delay
  cfblk3 : DiscreteFilter
  cfblk4 : Sin  TimeSource=Use external signal  SampleTime=0
  cfblk5 : PermuteDimensions
  cfblk6 : Sqrt  SaturateOnIntegerOverflow=on
  cfblk7 : Signum
  cfblk8 : Polyval  Coefs=[ +2.081618890e-019, -1.441693666e-014, +4.719686976e-010, -8.536869453e-006, +1.621573104e-001, -8.087801117e+001 ]
  cfblk9 : Constant  Value=[-500655078.326736]  SampleTime=1
  cfblk2 : Outport
  wires:
  cfblk6/1 -> cfblk3/1
  cfblk1/1 -> cfblk6/1
  cfblk8/1 -> cfblk2/1
  cfblk10/1 -> cfblk4/1
  cfblk5/1 -> cfblk7/1
  cfblk9/1 -> cfblk8/1
  cfblk7/1 -> cfblk13/1
  cfblk13/1 -> cfblk5/1

== system sampleModel7/cfblk383/cfblk16/cfblk7 ==
  cfblk1 : Inport
  cfblk11 : Inport  Port=2
  cfblk12 : Inport  Port=3
  cfblk13 : Inport  Port=4
  cfblk10 : Sum
  cfblk14 : Delay
  cfblk15 : Delay
  cfblk3 : Delay  DelayLengthSource=Input port
      settings: InputPortMap=u0,p1
  cfblk4 : simulink/Discrete/Transfer Fcn Lead or Lag  PoleZ=0.95  ZeroZ=0.75  ICPrevOutput=0.0  ICPrevInput=0.0  DoSatur=off
      settings: SourceProductBaseCode=SL
  cfblk5 : DiscreteIntegrator  SampleTime=-1  ICPrevOutput=DiscIntNeverNeededParam  ICPrevScaledInput=DiscIntNeverNeededParam
  cfblk6 : DiscreteTransferFcn
  cfblk7 : DotProduct  InputSameDT=on  OutDataTypeStr=Inherit: Inherit via internal rule
  cfblk8 : Gain  Gain=[469542065.360691]
  cfblk9 : MinMax  Function=max  Inputs=3
  cfblk2 : Outport
  wires:
  cfblk9/1 -> cfblk4/1
  cfblk1/1 -> cfblk5/1, cfblk9/3
  cfblk12/1 -> cfblk2/1
  cfblk6/1 -> cfblk7/1, cfblk3/2
  cfblk13/1 -> cfblk10/1
  cfblk5/1 -> cfblk10/2
  cfblk4/1 -> cfblk7/2
  cfblk11/1 -> cfblk6/1
  cfblk10/1 -> cfblk9/2
  cfblk3/1 -> cfblk8/1
  cfblk7/1 -> cfblk14/1
  cfblk14/1 -> cfblk9/1
  cfblk8/1 -> cfblk15/1
  cfblk15/1 -> cfblk3/1

== system sampleModel7/cfblk384/cfblk14/cfblk8 ==
  cfblk1 : Inport
  cfblk12 : Inport  Port=2
  cfblk13 : Inport  Port=3
  cfblk14 : Inport  Port=4
  cfblk15 : Inport  Port=5
  cfblk16 : Inport  Port=6
  cfblk17 : Inport  Port=7
  cfblk10 : Constant  Value=[286796668.630639]  SampleTime=1
  cfblk11 : Subsystem
  cfblk3 : DiscreteFir
  cfblk4 : simulink/Discrete/Transfer Fcn Lead or Lag  PoleZ=0.95  ZeroZ=0.75  ICPrevOutput=0.0  ICPrevInput=0.0  DoSatur=off
      settings: SourceProductBaseCode=SL
  cfblk5 : MinMax  Function=max
  cfblk6 : Sqrt  Operator=rSqrt  AlgorithmType=Newton-Raphson  SaturateOnIntegerOverflow=on
  cfblk7 : Product  Inputs=**
  cfblk8 : Gain  Gain=[983624891.515162]
  cfblk9 : Sqrt  SaturateOnIntegerOverflow=on
  cfblk2 : Outport
  wires:
  cfblk3/1 -> cfblk6/1
  cfblk16/1 -> cfblk7/1
  cfblk8/1 -> cfblk5/1
  cfblk15/1 -> cfblk2/1
  cfblk13/1 -> cfblk3/1
  cfblk9/1 -> cfblk11/1(cfblk1)
  cfblk7/1 -> cfblk8/1
  cfblk17/1 -> cfblk7/2
  cfblk10/1 -> cfblk4/1
  cfblk4/1 -> cfblk9/1
  cfblk5/1 -> cfblk11/2(cfblk8)
  cfblk14/1 -> cfblk11/3(cfblk9)
  cfblk1/1 -> cfblk11/4(cfblk10)

== system sampleModel7/cfblk388/cfblk18/cfblk7 ==
  cfblk1 : Inport
  cfblk10 : Inport  Port=2
  cfblk11 : Inport  Port=3
  cfblk12 : Inport  Port=4
  cfblk13 : Inport  Port=5
  cfblk14 : Inport  Port=6
  cfblk3 : simulink/Discrete/Transfer Fcn Lead or Lag  PoleZ=0.95  ZeroZ=0.75  ICPrevOutput=0.0  ICPrevInput=0.0  DoSatur=off
      settings: SourceProductBaseCode=SL
  cfblk4 : simulink/Discrete/Tapped Delay  vinit=0.0  samptime=-1  NumDelays=1  DelayOrder=Oldest  includeCurrent=off
  cfblk5 : Delay  ShowEnablePort=on
      settings: InputPortMap=u0,e6
  cfblk6 : Delay  ShowEnablePort=on
      settings: InputPortMap=u0,e6
  cfblk7 : Product  Inputs=*
  cfblk8 : Rounding
  cfblk9 : simulink/Math Operations/MinMax Running Resettable  Function=min  vinit=0.0
  cfblk2 : Outport
  wires:
  cfblk1/1 -> cfblk5/1
  cfblk12/1 -> cfblk3/1
  cfblk14/1 -> cfblk4/1
  cfblk11/1 -> cfblk7/1
  cfblk7/1 -> cfblk2/1
  cfblk13/1 -> cfblk5/2
  cfblk8/1 -> cfblk9/1
  cfblk4/1 -> cfblk6/1
  cfblk10/1 -> cfblk6/2
  cfblk5/1 -> cfblk9/2
  cfblk3/1 -> cfblk8/1

== system sampleModel7/cfblk396/cfblk6/cfblk13 ==
  cfblk1 : Inport
  cfblk14 : Inport  Port=2
  cfblk15 : Inport  Port=3
  cfblk16 : Inport  Port=4
  cfblk17 : Inport  Port=5
  cfblk10 : Trigonometry
  cfblk11 : Sqrt  SaturateOnIntegerOverflow=on
  cfblk12 : Constant  Value=[-819154569.005180]  SampleTime=1
  cfblk13 : Subsystem
  cfblk{3,7,18..19} (4 alike) : Delay
  cfblk4 : DiscreteZeroPole  Poles=[0 0.5]  Gain=1  SampleTime=-1
  cfblk5 : DiscreteFilter
  cfblk6 : DiscreteZeroPole  Poles=[0 0.5]  Gain=1  SampleTime=-1
  cfblk8 : DiscreteFilter
  cfblk9 : Assignment  DiagnosticForDimensions=Warning  IndexOptions=Index vector (dialog)  Indices=1  OutputSizes=1
  cfblk2 : Outport
  wires:
  cfblk6/1 -> cfblk8/1
  cfblk10/1 -> cfblk9/1
  cfblk1/1 -> cfblk10/1
  cfblk17/1 -> cfblk5/1
  cfblk9/1 -> cfblk4/1
  cfblk5/1 -> cfblk13/1(cfblk1)
  cfblk3/1 -> cfblk7/1
  cfblk4/1 -> cfblk13/2(cfblk10)
  cfblk16/1 -> cfblk3/1
  cfblk14/1 -> cfblk13/3(cfblk11)
  cfblk12/1 -> cfblk11/1
  cfblk11/1 -> cfblk13/4(cfblk12)
  cfblk15/1 -> cfblk2/1
  cfblk13/1(cfblk2) -> cfblk18/1
  cfblk18/1 -> cfblk9/2
  cfblk8/1 -> cfblk19/1
  cfblk19/1 -> cfblk6/1

== system sampleModel7/cfblk397/cfblk6/cfblk8 ==
  cfblk1 : Inport
  cfblk8 : Inport  Port=2
  cfblk9 : Inport  Port=3
  cfblk3 : simulink/Discrete/Tapped Delay  vinit=0.0  samptime=-1  NumDelays=1  DelayOrder=Oldest  includeCurrent=off
  cfblk4 : Product  Inputs=**
  cfblk5 : Constant  Value=[547468844.703990]  SampleTime=1
  cfblk6 : Constant  Value=[-826915916.448420]  SampleTime=1
  cfblk7 : Constant  Value=[308785418.195781]  SampleTime=1
  cfblk2 : Outport
  wires:
  cfblk6/1 -> cfblk2/1
  cfblk1/1 -> cfblk4/1
  cfblk7/1 -> cfblk3/1
  cfblk9/1 -> cfblk4/2

== system sampleModel7/cfblk399/cfblk15/cfblk6 ==
  cfblk1 : Inport
  cfblk9 : Inport  Port=2
  cfblk10 : Inport  Port=3
  cfblk11 : Inport  Port=4
  cfblk3 : Gain  Gain=[460023468.069956]
  cfblk4 : DotProduct  InputSameDT=on  OutDataTypeStr=Inherit: Inherit via internal rule
  cfblk5 : Sqrt  SaturateOnIntegerOverflow=on
  cfblk6 : simulink/Math Operations/Slider Gain  gain=1  low=0  high=2
  cfblk7 : Constant  Value=[-903081674.388361]  SampleTime=1
  cfblk8 : Subsystem
  cfblk2 : Outport
  wires:
  cfblk1/1 -> cfblk6/1
  cfblk7/1 -> cfblk4/1, cfblk8/5(cfblk13)
  cfblk6/1 -> cfblk8/1(cfblk1)
  cfblk4/1 -> cfblk5/1
  cfblk9/1 -> cfblk4/2, cfblk8/4(cfblk12)
  cfblk5/1 -> cfblk3/1, cfblk8/6(cfblk14)
  cfblk3/1 -> cfblk8/2(cfblk10)
  cfblk10/1 -> cfblk2/1
  cfblk11/1 -> cfblk8/3(cfblk11)

== system sampleModel7/cfblk402/cfblk13/cfblk6 ==
  cfblk1 : Inport
  cfblk8 : Inport  Port=2
  cfblk9 : Inport  Port=3
  cfblk10 : Inport  Port=4
  cfblk3 : ComplexToRealImag
  cfblk4 : Sqrt  Operator=rSqrt  AlgorithmType=Newton-Raphson  SaturateOnIntegerOverflow=on
  cfblk5 : Sum  Inputs=|++
  cfblk6 : simulink/Math Operations/MinMax Running Resettable  Function=min  vinit=0.0
  cfblk7 : Constant  Value=[-433139034.806955]  SampleTime=1
  cfblk2 : Outport
  wires:
  cfblk4/1 -> cfblk5/1
  cfblk3/1 -> cfblk6/1
  cfblk1/1 -> cfblk4/1
  cfblk10/1 -> cfblk5/2
  cfblk9/1 -> cfblk2/1
  cfblk5/1 -> cfblk6/2
  cfblk8/1 -> cfblk3/1
